simulink model "LOSdemo2"  (R2016b)
settings: Solver=ode1  StartTime=0.0  StopTime=300  FixedStep=0.01  RelTol=1e-3
libraries: simulink x2
settings Model: Creator=qys  LastModifiedBy=qys

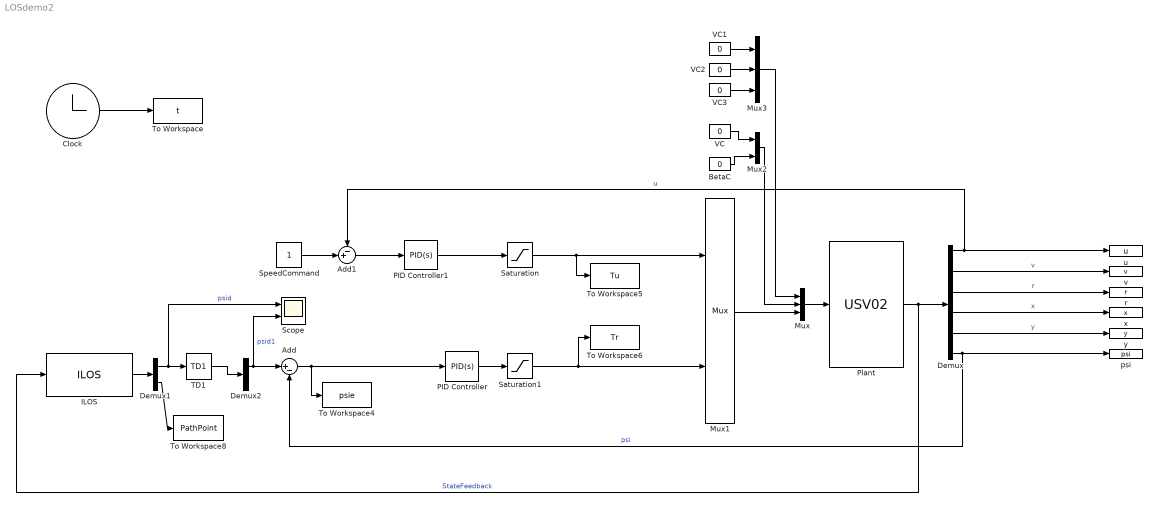
== system LOSdemo2 ==
  Add : Sum  Inputs=|+-
  Add1 : Sum  Inputs=-+|
  BetaC : Constant  Value=0
  Clock : Clock
  Demux : Demux  Outputs=6
  Demux1 : Demux  Outputs=2
  Demux2 : Demux  Outputs=2
  ILOS : S-Function  FunctionName=ILOS  SFunctionDeploymentMode=off  EnableBusSupport=off
  Mux : Mux  Inputs=[3 2 2]
  Mux1 : Mux  Inputs=2
  Mux2 : Mux  Inputs=2
  Mux3 : Mux  Inputs=3
  PID Controller : simulink/Continuous/PID Controller  Controller=PID  TimeDomain=Continuous-time  SampleTime=-1  IntegratorMethod=Forward Euler  FilterMethod=Forward Euler  Form=Parallel  UseFilter=on  ControllerParametersSource=internal  P=60  I=0  D=40  N=100  InitialConditionSource=internal  InitialConditionForIntegrator=0  InitialConditionForFilter=0  ExternalReset=none  LimitOutput=off  UpperSaturationLimit=5  LowerSaturationLimit=-5  LinearizeAsGain=on  AntiWindupMode=none  Kb=1  TrackingMode=off  Kt=1  PParamMin=[]  PParamMax=[]  IParamMin=[]  IParamMax=[]  DParamMin=[]  DParamMax=[]  NParamMin=[]  NParamMax=[]  KbParamMin=[]  KbParamMax=[]  KtParamMin=[]  KtParamMax=[]  POutMin=[]  POutMax=[]  IOutMin=[]  IOutMax=[]  DOutMin=[]  DOutMax=[]  NOutMin=[]  NOutMax=[]  KbOutMin=[]  KbOutMax=[]  KtOutMin=[]  KtOutMax=[]  IntegratorOutMin=[]  IntegratorOutMax=[]  FilterOutMin=[]  FilterOutMax=[]  SumOutMin=[]  SumOutMax=[]  SumI1OutMin=[]  SumI1OutMax=[]  SumI2OutMin=[]  SumI2OutMax=[]  SumI3OutMin=[]  SumI3OutMax=[]  SumDOutMin=[]  SumDOutMax=[]  SaturationOutMin=[]  SaturationOutMax=[]  IntegratorContinuousStateAttributes=''  IntegratorStateMustResolveToSignalObject=off  IntegratorRTWStateStorageClass=Auto  FilterContinuousStateAttributes=''  FilterStateMustResolveToSignalObject=off  FilterRTWStateStorageClass=Auto  DifferentiatorICPrevScaledInput=0  DifferentiatorOutMin=[]  DifferentiatorOutMax=[]
  PID Controller1 : simulink/Continuous/PID Controller  Controller=PID  TimeDomain=Continuous-time  SampleTime=-1  IntegratorMethod=Forward Euler  FilterMethod=Forward Euler  Form=Parallel  UseFilter=on  ControllerParametersSource=internal  P=20  I=1  D=8  N=100  InitialConditionSource=internal  InitialConditionForIntegrator=0  InitialConditionForFilter=0  ExternalReset=none  LimitOutput=off  UpperSaturationLimit=10  LowerSaturationLimit=-10  LinearizeAsGain=on  AntiWindupMode=none  Kb=1  TrackingMode=off  Kt=1  PParamMin=[]  PParamMax=[]  IParamMin=[]  IParamMax=[]  DParamMin=[]  DParamMax=[]  NParamMin=[]  NParamMax=[]  KbParamMin=[]  KbParamMax=[]  KtParamMin=[]  KtParamMax=[]  POutMin=[]  POutMax=[]  IOutMin=[]  IOutMax=[]  DOutMin=[]  DOutMax=[]  NOutMin=[]  NOutMax=[]  KbOutMin=[]  KbOutMax=[]  KtOutMin=[]  KtOutMax=[]  IntegratorOutMin=[]  IntegratorOutMax=[]  FilterOutMin=[]  FilterOutMax=[]  SumOutMin=[]  SumOutMax=[]  SumI1OutMin=[]  SumI1OutMax=[]  SumI2OutMin=[]  SumI2OutMax=[]  SumI3OutMin=[]  SumI3OutMax=[]  SumDOutMin=[]  SumDOutMax=[]  SaturationOutMin=[]  SaturationOutMax=[]  IntegratorContinuousStateAttributes=''  IntegratorStateMustResolveToSignalObject=off  IntegratorRTWStateStorageClass=Auto  FilterContinuousStateAttributes=''  FilterStateMustResolveToSignalObject=off  FilterRTWStateStorageClass=Auto  DifferentiatorICPrevScaledInput=0  DifferentiatorOutMin=[]  DifferentiatorOutMax=[]
  Plant : S-Function  FunctionName=USV02  SFunctionDeploymentMode=off  EnableBusSupport=off
  Saturation : Saturate  UpperLimit=10  LowerLimit=0
  Saturation1 : Saturate  UpperLimit=5  LowerLimit=-5
  Scope : Scope  NumInputPorts=2
  SpeedCommand : Constant
  TD1 : S-Function  FunctionName=TD1  SFunctionDeploymentMode=off  EnableBusSupport=off
  To Workspace : ToWorkspace  VariableName=t  SampleTime=-1
  To Workspace4 : ToWorkspace  VariableName=psie  SampleTime=-1
  To Workspace5 : ToWorkspace  VariableName=Tu  SampleTime=-1
  To Workspace6 : ToWorkspace  VariableName=Tr  SampleTime=-1
  To Workspace8 : ToWorkspace  VariableName=PathPoint  SampleTime=-1
  VC{,1..3} (4 alike) : Constant  Value=0
  psi : ToWorkspace  VariableName=psi  SampleTime=-1
  r : ToWorkspace  VariableName=r  SampleTime=-1
  u : ToWorkspace  VariableName=u  SampleTime=-1
  v : ToWorkspace  VariableName=v  SampleTime=-1
  x : ToWorkspace  VariableName=x  SampleTime=-1
  y : ToWorkspace  VariableName=y  SampleTime=-1
  wires:
  Plant/1 -> ILOS/1, Demux/1  "StateFeedback"
  Mux/1 -> Plant/1
  Mux2/1 -> Mux/2
  Mux1/1 -> Mux/3
  Mux3/1 -> Mux/1
  PID Controller1/1 -> Saturation/1
  PID Controller/1 -> Saturation1/1
  VC/1 -> Mux2/1
  BetaC/1 -> Mux2/2
  VC1/1 -> Mux3/1
  VC2/1 -> Mux3/2
  VC3/1 -> Mux3/3
  Add/1 -> PID Controller/1, To Workspace4/1
  Add1/1 -> PID Controller1/1
  Demux/1 -> Add1/1, u/1  "u"
  SpeedCommand/1 -> Add1/2
  Clock/1 -> To Workspace/1
  Demux/6 -> Add/2, psi/1  "psi"
  ILOS/1 -> Demux1/1
  Demux1/1 -> Scope/1, TD1/1  "psid"
  Demux1/2 -> To Workspace8/1
  Saturation1/1 -> Mux1/2, To Workspace6/1
  Saturation/1 -> To Workspace5/1, Mux1/1
  Demux/4 -> x/1  "x"
  Demux/5 -> y/1  "y"
  Demux/3 -> r/1  "r"
  Demux/2 -> v/1  "v"
  TD1/1 -> Demux2/1
  Demux2/1 -> Scope/2, Add/1  "psid1"
